simulink model "IMRPROTest"  (R2020b)
settings: Solver=FixedStepAuto  StartTime=0.0  StopTime=100  RelTol=1e-3  EnableMultiTasking=on
InitFcn:
  | load('BusDefinitions.mat')
  | codertarget.parrot.internal.checkImageBlocks(gcs)
undefined symbols (not defined in the file or in its folder): codertarget, gray, Ts
libraries: parrotlib x1
settings Model: ExtModeTrigDuration=80  ExtModeArchiveDirName=/Users/NathanDurocher/Desktop/test  ExtModeLogAll=off  Creator=NathanDurocher  LastModifiedBy=NathanDurocher
settings SolverCC: PositivePriorityOrder=on
settings OptimizationCC: PassReuseOutputArgsThreshold=0  MaxStackSize=64
settings DebuggingCC: ParameterTunabilityLossMsg=error  ArithmeticOperatorsInVariantConditions=warning
settings HardwareCC: ProdBitPerPointer=32  ProdBitPerSizeT=32  ProdBitPerPtrDiffT=32  ProdLargestAtomicInteger=Long  ProdWordSize=32  ProdHWDeviceType=ARM Compatible->ARM 9  UseEmbeddedCoderFeatures=off
settings SFSimCC: SimUseLocalCustomCode=off
settings RTWCC: Description=Embedded Coder  SystemTargetFile=ert.tlc  HardwareBoard=PARROT Mambo  TemplateMakefile=ert_default_tmf  GenerateReport=on  RTWUseLocalCustomCode=off  Toolchain=Sourcery G++ Lite GNU Toolchain for Drones  LaunchReport=on
settings CodeAppCC: ForceParamTrailComments=on  OperatorAnnotations=on  StateflowObjectComments=on
settings ERTTargetCC: ERTCustomFileBanners=off  SupportContinuousTime=on  SupportNonInlinedSFcns=on  RemoveResetFunc=off  ModelStepFunctionPrototypeControlCompliant=off

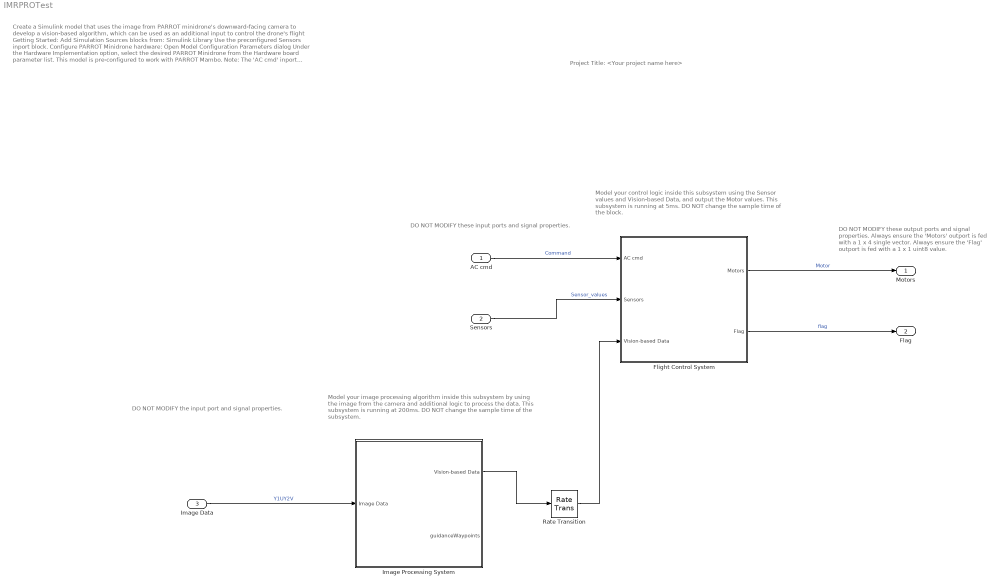
== system IMRPROTest ==
  note: Model your control logic inside this subsystem
      | using the Sensor values and Vision-based Data,
      | and output the Motor values.
      | This subsystem is running at 5ms.
      | DO NOT change the sample time of the block.
  note: DO NOT MODIFY these output ports
      | and signal properties.
      |
      |
      |
      |
      |
      | Always ensure the 'Motors' outport
      | is fed with a 1 x 4 single vector.
      |
      |
      |
      |
      |
      | Always ensure the 'Flag' outport is
      | fed with a 1 x 1 uint8 value.
  note: DO NOT MODIFY these input
      | ports and signal properties.
  note: Create a Simulink model that uses the image from PARROT minidrone's downward-facing camera to develop a vision-based algorithm, which can be used as an additional input to control the drone's flight
      |
      | Getting Started:
      |
      | Add Simulation Sources blocks from:
      | Simulink Library
      | Use the preconfigured Sensors inport block.
      |
      | Configure PARROT Minidrone hardware:
      |
      | Open Model Configuration Parameters dialog
      |
      | Under the Hardware Implementation option, select the desired
      | PARROT Minidrone from the Hardware board parameter list.
      |
      | This model is pre-configured to work with PARROT Mambo.
      |
      | Note:
      |
      | The 'AC cmd' inport contains the position and orientation reference signals information.
      | The 'Sensors' inport contains data from accelerometer, gyroscope, ultrasonic, pressure and optical flow data.
      | The 'Flag' outport can be used to model an error condition which stops the drone.
      | The 'Motors' outport is fed with the speed values of the 4 motors.
      | The 'Image Data' inport of the Image Processing System represents the image obtained from the downward-facing camera of PARROT minidrone, in Y1UY2V format.
      | The 'Vision-based Data' inport of Flight Control System represents the data obtained from the image processing algorithm inside the Image Processing System.
      | Learn more:
      |
      | Simulink Subsystem
      | Simulink Buses
  note: Project Title: <Your project name here>
  note: DO NOT MODIFY the input port and
      | signal properties.
  note: Model your image processing algorithm inside this
      | subsystem by using the image from the camera
      | and additional logic to process the data.
      | This subsystem is running at 200ms.
      | DO NOT change the sample time of the subsystem.
  AC cmd : Inport  OutDataTypeStr=Bus: CommandBus  BusOutputAsStruct=on
  Sensors : Inport  Port=2  OutDataTypeStr=Bus: SensorsBus  BusOutputAsStruct=on
  Image Data : Inport  Tag=IP_IN  InitFcn=codertarget.parrot.internal.inportCallback(gcb);  Port=3  OutDataTypeStr=uint8  PortDimensions=[4 9600]  BusOutputAsStruct=on
  Flight Control System : Subsystem  InitFcn=codertarget.parrot.internal.fcsSubsystemCallback(gcb);  TreatAsAtomicUnit=on  SystemSampleTime=Ts
  Image Processing System : Subsystem  Tag=IP_SUB  InitFcn=codertarget.parrot.internal.ipSubsystemCallback(gcb);  TreatAsAtomicUnit=on  SystemSampleTime=40*Ts  RTWFcnName=ImageFunction
      settings: RTWSystemCode=Inline  RTWFcnNameOpts=User specified
  Rate Transition : RateTransition  Deterministic=off
  Motors : Outport  OutDataTypeStr=single  PortDimensions=[1 4]  VectorParamsAs1DForOutWhenUnconnected=off
  Flag : Outport  Port=2  OutDataTypeStr=uint8  PortDimensions=1  VectorParamsAs1DForOutWhenUnconnected=off
  wires:
  Flight Control System/1(Motors) -> Motors/1  "Motor"
  AC cmd/1 -> Flight Control System/1(AC cmd)  "Command"
  Sensors/1 -> Flight Control System/2(Sensors)  "Sensor_values"
  Flight Control System/2(Flag) -> Flag/1  "flag"
  Image Data/1 -> Image Processing System/1(Image Data)  "Y1UY2V"
  Rate Transition/1 -> Flight Control System/3(" Vision-based Data")
  Image Processing System/1(" Vision-based Data") -> Rate Transition/1

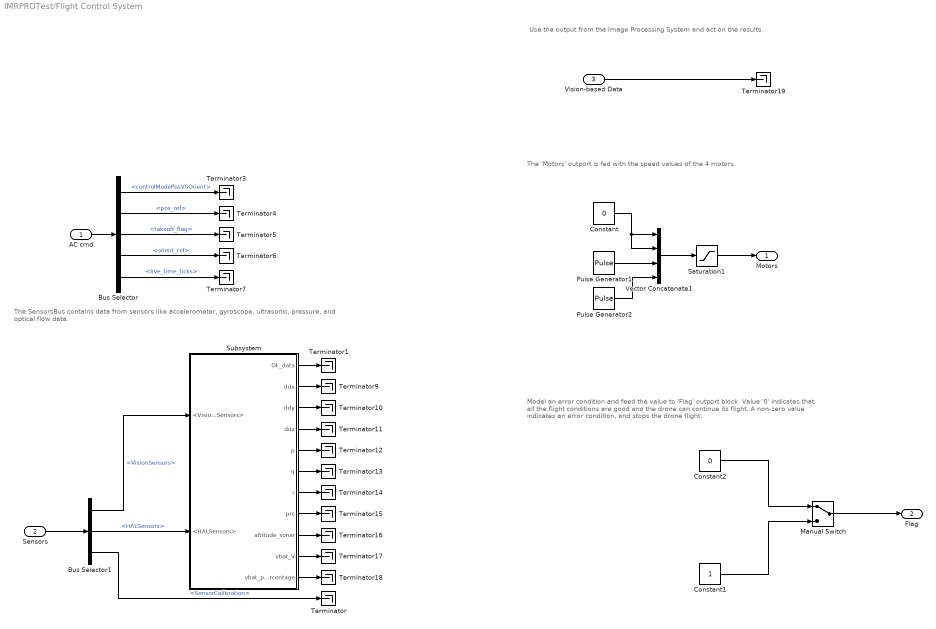
== system IMRPROTest/Flight Control System ==
  note: The 'Motors' outport is fed with the speed values of the 4 motors.
  note: Model an error condition and feed the value to 'Flag' outport block.
      | Value '0' indicates that all the flight conditions are good and the drone
      | can continue its flight.
      | A non-zero value indicates an error condition, and stops the drone
      | flight.
  note: The SensorsBus contains data from sensors like
      | accelerometer, gyroscope, ultrasonic, pressure,
      | and optical flow data.
  note: Use the output from the Image Processing System and act on the
      | results.
  AC cmd : Inport
  Sensors : Inport  Port=2
  " Vision-based Data" : Inport  Port=3
  Bus Selector : BusSelector  OutputSignals=controlModePosVSOrient,pos_ref,takeoff_flag,orient_ref,live_time_ticks
  Bus Selector1 : BusSelector  OutputSignals=VisionSensors,HALSensors,SensorCalibration
  Constant : Constant  Value=0
  Constant1 : Constant  OutDataTypeStr=uint8
  Constant2 : Constant  Value=0  OutDataTypeStr=uint8
  Manual Switch : ManualSwitch
  Pulse Generator1 : DiscretePulseGenerator  Amplitude=400  Period=800  PulseWidth=400  SampleTime=Ts
  Pulse Generator2 : DiscretePulseGenerator  Amplitude=400  Period=800  PulseWidth=400  PhaseDelay=400  SampleTime=Ts
  Saturation1 : Saturate  UpperLimit=500  LowerLimit=0  OutDataTypeStr=single
  Subsystem : Subsystem
  Terminator{,1,3..7,9..19} (18 alike) : Terminator
  Vector Concatenate1 : Concatenate  NumInputs=4
  Motors : Outport  VectorParamsAs1DForOutWhenUnconnected=off
  Flag : Outport  Port=2  VectorParamsAs1DForOutWhenUnconnected=off
  wires:
  AC cmd/1 -> Bus Selector/1
  Sensors/1 -> Bus Selector1/1
  Bus Selector/1 -> Terminator3/1  "<controlModePosVSOrient>"
  Bus Selector/2 -> Terminator4/1  "<pos_ref>"
  Bus Selector/3 -> Terminator5/1  "<takeoff_flag>"
  Bus Selector/4 -> Terminator6/1  "<orient_ref>"
  Bus Selector/5 -> Terminator7/1  "<live_time_ticks>"
  Manual Switch/1 -> Flag/1
  Constant2/1 -> Manual Switch/1
  Constant1/1 -> Manual Switch/2
  Vector Concatenate1/1 -> Saturation1/1
  Pulse Generator2/1 -> Vector Concatenate1/4
  Saturation1/1 -> Motors/1
  Bus Selector1/1 -> Subsystem/1(<VisionSensors>)  "<VisionSensors>"
  Bus Selector1/2 -> Subsystem/2(<HALSensors>)  "<HALSensors>"
  Bus Selector1/3 -> Terminator/1  "<SensorCalibration>"
  Subsystem/1(OF_data) -> Terminator1/1
  Subsystem/2(ddx) -> Terminator9/1
  Subsystem/3(ddy) -> Terminator10/1
  Subsystem/4(ddz) -> Terminator11/1
  Subsystem/5(p) -> Terminator12/1
  Subsystem/7(r) -> Terminator14/1
  Subsystem/8(prs) -> Terminator15/1
  Subsystem/9(altitude_sonar) -> Terminator16/1
  Subsystem/10(vbat_V) -> Terminator17/1
  Subsystem/11(vbat_percentage) -> Terminator18/1
  Subsystem/6(q) -> Terminator13/1
  Constant/1 -> Vector Concatenate1/2, Vector Concatenate1/1
  " Vision-based Data"/1 -> Terminator19/1
  Pulse Generator1/1 -> Vector Concatenate1/3

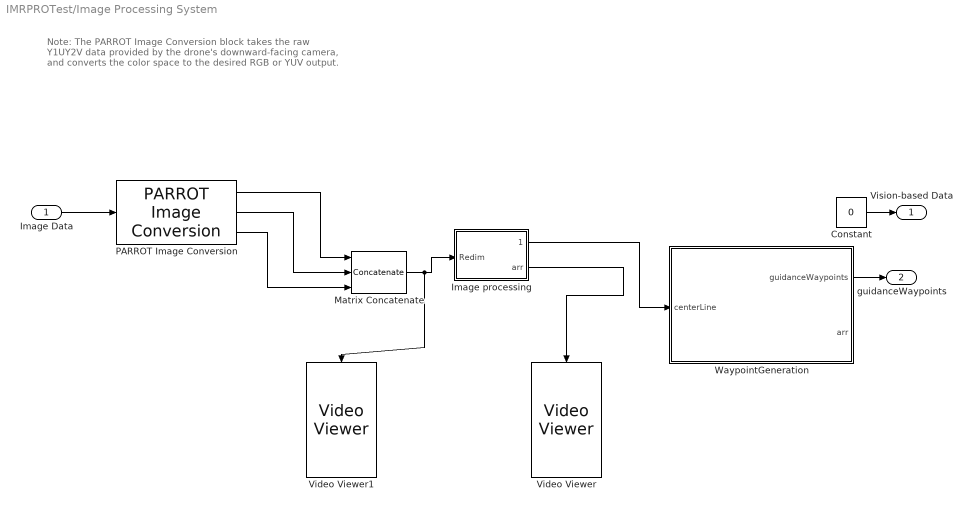
== system IMRPROTest/Image Processing System ==
  note: Note:
      |
      | The PARROT Image Conversion block takes the raw Y1UY2V data provided by the drone's downward-facing camera, and converts the color space to the desired RGB or YUV output.
  Image Data : Inport
  Constant : Constant  Value=0
  Image processing : MATLAB Function  TreatAsAtomicUnit=on
  Matrix Concatenate : Concatenate  NumInputs=3  Mode=Multidimensional array  ConcatenateDimension=3
  PARROT Image Conversion : parrotlib/PARROT Image Conversion  Tag=IP_FORMAT  ImageFormat=RGB  R=on  Y=on  G=on  U=on  B=on  V=on
      settings: SourceProductName=Simulink Support Package for Parrot Minidrones
  Video Viewer : VideoViewer  ExtModeUploadOption=log  colormapValue=gray(256)  FigPos=[319 856 418 304]
  Video Viewer1 : VideoViewer  ExtModeUploadOption=log  colormapValue=gray(256)  FigPos=[738 856 418 304]
  WaypointGeneration : MATLAB Function  TreatAsAtomicUnit=on
  " Vision-based Data" : Outport  VectorParamsAs1DForOutWhenUnconnected=off
  guidanceWaypoints : Outport  Port=2
  wires:
  Image Data/1 -> PARROT Image Conversion/1
  Constant/1 -> " Vision-based Data"/1
  Image processing/1(centerLine) -> WaypointGeneration/1(centerLine)
  PARROT Image Conversion/2 -> Matrix Concatenate/2
  PARROT Image Conversion/1 -> Matrix Concatenate/1
  Image processing/2(arr) -> Video Viewer/1
  PARROT Image Conversion/3 -> Matrix Concatenate/3
  WaypointGeneration/1(guidanceWaypoints) -> guidanceWaypoints/1
  Matrix Concatenate/1 -> Video Viewer1/1, Image processing/1(Redim)

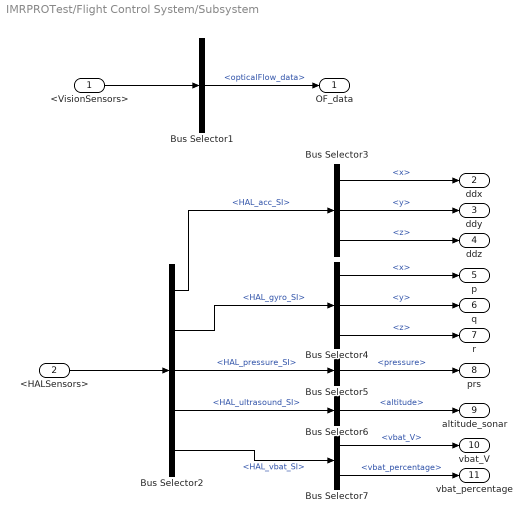
== system IMRPROTest/Flight Control System/Subsystem ==
  <VisionSensors> : Inport
  <HALSensors> : Inport  Port=2
  Bus Selector1 : BusSelector  OutputSignals=opticalFlow_data
  Bus Selector2 : BusSelector  OutputSignals=HAL_acc_SI,HAL_gyro_SI,HAL_pressure_SI,HAL_ultrasound_SI,HAL_vbat_SI
  Bus Selector3 : BusSelector  OutputSignals=x,y,z
  Bus Selector4 : BusSelector  OutputSignals=x,y,z
  Bus Selector5 : BusSelector  OutputSignals=pressure
  Bus Selector6 : BusSelector  OutputSignals=altitude
  Bus Selector7 : BusSelector  OutputSignals=vbat_V,vbat_percentage
  OF_data : Outport  VectorParamsAs1DForOutWhenUnconnected=off
  ddx : Outport  Port=2  VectorParamsAs1DForOutWhenUnconnected=off
  ddy : Outport  Port=3  VectorParamsAs1DForOutWhenUnconnected=off
  ddz : Outport  Port=4  VectorParamsAs1DForOutWhenUnconnected=off
  p : Outport  Port=5  VectorParamsAs1DForOutWhenUnconnected=off
  q : Outport  Port=6  VectorParamsAs1DForOutWhenUnconnected=off
  r : Outport  Port=7  VectorParamsAs1DForOutWhenUnconnected=off
  prs : Outport  Port=8  VectorParamsAs1DForOutWhenUnconnected=off
  altitude_sonar : Outport  Port=9  VectorParamsAs1DForOutWhenUnconnected=off
  vbat_V : Outport  Port=10  VectorParamsAs1DForOutWhenUnconnected=off
  vbat_percentage : Outport  Port=11  VectorParamsAs1DForOutWhenUnconnected=off
  wires:
  <VisionSensors>/1 -> Bus Selector1/1
  <HALSensors>/1 -> Bus Selector2/1
  Bus Selector1/1 -> OF_data/1  "<opticalFlow_data>"
  Bus Selector2/1 -> Bus Selector3/1  "<HAL_acc_SI>"
  Bus Selector2/2 -> Bus Selector4/1  "<HAL_gyro_SI>"
  Bus Selector2/3 -> Bus Selector5/1  "<HAL_pressure_SI>"
  Bus Selector2/4 -> Bus Selector6/1  "<HAL_ultrasound_SI>"
  Bus Selector2/5 -> Bus Selector7/1  "<HAL_vbat_SI>"
  Bus Selector3/1 -> ddx/1  "<x>"
  Bus Selector3/2 -> ddy/1  "<y>"
  Bus Selector3/3 -> ddz/1  "<z>"
  Bus Selector4/2 -> q/1  "<y>"
  Bus Selector4/1 -> p/1  "<x>"
  Bus Selector4/3 -> r/1  "<z>"
  Bus Selector5/1 -> prs/1  "<pressure>"
  Bus Selector6/1 -> altitude_sonar/1  "<altitude>"
  Bus Selector7/1 -> vbat_V/1  "<vbat_V>"
  Bus Selector7/2 -> vbat_percentage/1  "<vbat_percentage>"

== matlab function IMRPROTest/Image Processing System/WaypointGeneration ==
  data: centerLine input; guidanceWaypoints output size=[2,2]; arr output
function [guidanceWaypoints, arr] = WaypointGenerationDebug(centerLine)
if coder.target('MATLAB')
    clear;
    clc;
    close all;
    centerLine = readmatrix('waypoints.txt')
    pic = imread('waypoints.png');
    figure('Name', 'Read path');
    imshow(pic);
    impixelinfo;
    img = uint8(zeros(size(pic,1),size(pic,2)));
    arr = uint8(zeros(size(pic,1),size(pic,2)));
else
    arr = uint8(zeros(120,160));
    waypointsInfront=[];
end

guidanceWaypoints = [60, 80; 60, 80];
[arr, waypoints]=pointsToCenterLine(centerLine,arr);
% [~, waypoints]=pointsToCenterLine(centerLine,[]);
list= single(waypoints);

coder.varsize('sortedWaypoints')
sortedWaypoints = zeros(size(list,1),4);
for i=1:size(list,1)
   [arcos,D]=getAngleToImgCenter([list(i,1), list(i,2)]);
    sortedWaypoints(i,:) = [list(i,:),arcos,D];
end
if(size(sortedWaypoints,1)==0)
    return
end
[v,i]=min(sortedWaypoints(:,4));
% We got a list of sorted waypoints, but we don't know whats up and down...
% Straight up gives us an angle of 1, straigt down of -1, so let's go in
% this direction where we get the higher number of the next couple of
% angles
elementsUpwards=(size(sortedWaypoints,1)-i);
upwards=sum(sortedWaypoints(i:i+elementsUpwards,3))/(elementsUpwards+1);
elementsDownwards=i;
downwards=sum(sortedWaypoints(1:i,3))/elementsDownwards;
if(upwards>downwards)
    waypointsInfront = sortedWaypoints(i:size(sortedWaypoints,1),:);
else
    waypointsInfront = sortedWaypoints(i:-1:1,:);
end
l = size(waypointsInfront,1);

if (l-20) >= 1
    dtoplist = norm(waypointsInfront(1,1:2)-[60,80]);
    dbottomlist = norm(waypointsInfront(l,1:2)-[60,80]);
    if dbottomlist > dtoplist
        guidanceWaypoints =[waypointsInfront(l-20,1:2);waypointsInfront(l,1:2)];
    else 
        guidanceWaypoints =[waypointsInfront(1,1:2);waypointsInfront(21,1:2)];
    end
end
if coder.target('MATLAB')
    idx=sub2ind(size(img),waypointsInfront(:,1), waypointsInfront(:,2));
    img(idx)=255;
    
    figure('Name','Path to follow');
    imshow(img);
    impixelinfo;
end

== matlab function IMRPROTest/Image Processing System/Image processing ==
  data: centerLine output double size=[4,2]; Redim input; arr output
function [centerLine,arr] = fcn(Redim)
if coder.target('MATLAB')
    clear;
    clc;
    close all;
%     pic = imread("TestImages/Mambo_2021-05-21T190412+0200_.jpg");
    pic = imread("TestImages/FailCorner1.png");
%     imshow(pic);
else
    pic=Redim;
end

arr = uint8(zeros(size(pic,1),size(pic,2)));
% coder.varsize('centerLine',[4,2], [4,2]);
coder.varsize('centerLine');
centerLine = double([4,2]);
lineWidthInPixel=50;
% pic = imread("goal.jpg");
% lineWidthInPixel=110;
BW = maskImageRGB(pic);
BW=bwmorph(BW, 'skel', 50);

[H,theta,rho] = hough(BW);

nHoodSize = int32(size(H)/50);
nHoodSize = double(nHoodSize);
P = houghpeaks(H,20,'threshold',ceil(0.1*max(H(:))), 'NHoodSize', [1,1]);
x = theta(P(:,2));
y = rho(P(:,1));


lines = houghlines(BW,theta,rho,P,'FillGap',lineWidthInPixel*2/3,'MinLength',lineWidthInPixel);
if isempty(lines)
    return
end



coder.varsize('c_lines');

c_linesTemp = struct2cell(lines);
cLinesSize = size(c_linesTemp,3);
c_lines = cell(5,1,cLinesSize);
for idx = 1:cLinesSize
    c_lines{1,1,idx} = c_linesTemp{1,idx};
    c_lines{2,1,idx} = c_linesTemp{2,idx};
    c_lines{3,1,idx} = c_linesTemp{3,idx};
    c_lines{4,1,idx} = c_linesTemp{4,idx};
    c_lines{5,1,idx} = 0;
end
if coder.target('MATLAB')
    figure
    imshow(BW)
    hold on
end
max_len = 0;
for k = 1:length(lines)
   xy = [lines(k).point1; lines(k).point2];
   if coder.target('MATLAB')
       plot(xy(:,1),xy(:,2),'LineWidth',2,'Color','green');

       % Plot beginnings and ends of lines
       plot(xy(1,1),xy(1,2),'x','LineWidth',2,'Color','yellow');
       plot(xy(2,1),xy(2,2),'x','LineWidth',2,'Color','red');
       impixelinfo
   end

   % Determine the endpoints of the longest line segment
   len = norm(c_lines{1,1,k} - c_lines{2,1,k});
   if ( len > max_len)
      max_len = len;
      xy_long = xy;
   end
end

%% Test
uniqueTheta = unique([c_lines{3,:,:}]','rows');
concLines = concatAllLines(c_lines, lineWidthInPixel);
% if(size(concLines,2)==1)
%     %looks like we only found one line, most likely because we're at the
%     %starting point or infront of us is the goal, so let's remove the cross
%     %section manually...
%     s = size(c_lines,3);
% %     coder.varsize('linesWithoutOutlier')
%     coder.varsize('isNoOutlier')
%     coder.varsize('temp')
%     isNoOutlier = not(isoutlier([c_lines{3,1,1:s}]));
%     cellSize_ = sum(isNoOutlier==1,2);
%     cellSize = cellSize_(1);
%     linesWithoutOutlier=cell(5,1,cellSize);
%     outlierIdx = 1;
%     for idx=1:cellSize
%             while(isNoOutlier(outlierIdx)==0)
%                 outlierIdx = outlierIdx + 1;
%             end       
%             linesWithoutOutlier{1,1,idx} = c_lines{1,outlierIdx};
%             linesWithoutOutlier{2,1,idx} = c_lines{2,outlierIdx};
%             linesWithoutOutlier{3,1,idx} = c_lines{3,outlierIdx};
%             linesWithoutOutlier{4,1,idx} = c_lines{4,outlierIdx};
%             linesWithoutOutlier{5,1,idx} = c_lines{5,outlierIdx};
%             outlierIdx = outlierIdx + 1;
%         
%     end
%     concLines = concatAllLines(linesWithoutOutlier, lineWidthInPixel);
% end

% if size(concLines,2)==2
%     line1=splitLineInSegments(concLines{1});
%     line2=splitLineInSegments(concLines{2});
% elseif(size(concLines,2)==3)
%         lineS1 = splitLineInSegments(concLines{1});
%         lineS2 = splitLineInSegments(concLines{2});
%         lineS3 = splitLineInSegments(concLines{3});
%         if(size(lineS1,1)==4)
%             line1=lineS1;
%             if((lineS1(1,3)^2-lineS2(1,3)^2)<(lineS1(1,3)^2-lineS3(1,3)^2))
%                 line2 = [lineS2;lineS3];
%             else
%                 line2 = [lineS3;lineS2];
%             end
%         elseif(size(lineS2,1)==4)
%             line1 = lineS2;
%             if((lineS2(1,3)^2-lineS1(1,3)^2)<(lineS2(1,3)^2-lineS3(1,3)^2))
%                 line2 = [lineS1;lineS3];
%             else
%                 line2 = [lineS3;lineS1];
%             end
%         elseif(size(lineS3,1)==4)
%             line1 = lineS3;
%             if((lineS3(1,3)^2-lineS1(1,3)^2)<(lineS3(1,3)^2-lineS2(1,3)^2))
%                 line2 = [lineS1;lineS2];
%             else
%                 line2 = [lineS2;lineS1];
%             end
%         else
%             %just take the two longest segments and hope for the best...
%             [v,i]=min([pdist(lineS1(:,1:2)), pdist(lineS2(:,1:2)), pdist(lineS3(:,1:2))]);
%             switch(i)
%                 case 1 
%                     line1= lineS2;
%                     line2= lineS3;
%                 case 2
%                     line1 = lineS1;
%                     line2 = lineS3;
%                 case 3
%                     line1 = lineS1;
%                     line2 = lineS2;
%             end
%         end
% else
%     fprintf("Could not detect the centerLine")
%     return
% end
if(size(concLines,1)>=1)
    splitLines = splitLineInSegments(concLines{1})
    centerLine = splitLines(:,1:2);
    centerLine = orderCenterline(centerLine);
end
%% Looks like the split up did not work properly, let's remove the shortest segment and hope for the best...
% if(size(line1,1)~=size(line2,1))
%     while(size(line1,1)>size(line2,1))
%         [val,idx]=min(line1(:,4));
%         line1(idx:idx+1,:)=[];
%     end
%     while(size(line2,1)>size(line1,1))
%         [val,idx]=min(line2(:,4));
%         line2(idx:idx+1,:)=[];
%     end
% end
% for i=1:2:size(line1,1)
%     xDiff = abs(line1(i,1)-line1(i+1,1));
%     yDiff = abs(line1(i,2)-line1(i+1,2));
%     if(xDiff>yDiff)
%         if(line1(i,1)>line1(i+1,1))
%             line1([i,i+1],:)=line1([i+1,i],:);
%         end
%         if(line2(i,1)>line2(i+1,1))
%             line2([i,i+1],:)=line2([i+1,i],:);
%         end
%     else
%          if(line1(i,2)>line1(i+1,2))
%             line1([i,i+1],:)=line1([i+1,i],:);
%         end
%         if(line2(i,2)>line2(i+1,2))
%             line2([i,i+1],:)=line2([i+1,i],:);
%         end
%     end
% end
% centerLine = floor((line1(:,1:2)+line2(:,1:2))./2);
% centerLine = orderCenterline(centerLine);
[arr, waypoints] = pointsToCenterLine(centerLine, arr);

if coder.target('MATLAB')
    figure;
    imshow(arr);
    imwrite(arr, 'waypoints.png');
    writematrix(centerLine, 'waypoints.txt')
%     waypointFile = fopen('waypoints.pmc', 'w')
%     fprintf(waypointFile,centerLine);
%     WaypointGenerationDebug(centerLine);
end
